simulink model "Force_Jawwad"  (R2023a)
settings: Solver=VariableStepAuto  StartTime=0.0  StopTime=5  RelTol=1e-3
undefined symbols (not defined in the file): fd, Kd, Kf, Ki, Kp, Md, parms
settings Model: Creator=uzair  LastModifiedBy=syedj
settings OptimizationCC: ReuseModelBlockBuffer=off

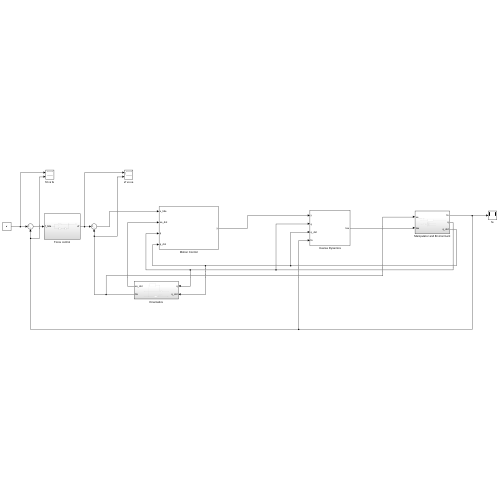
[thumbnail: Simulink's stored preview of the top-level diagram]
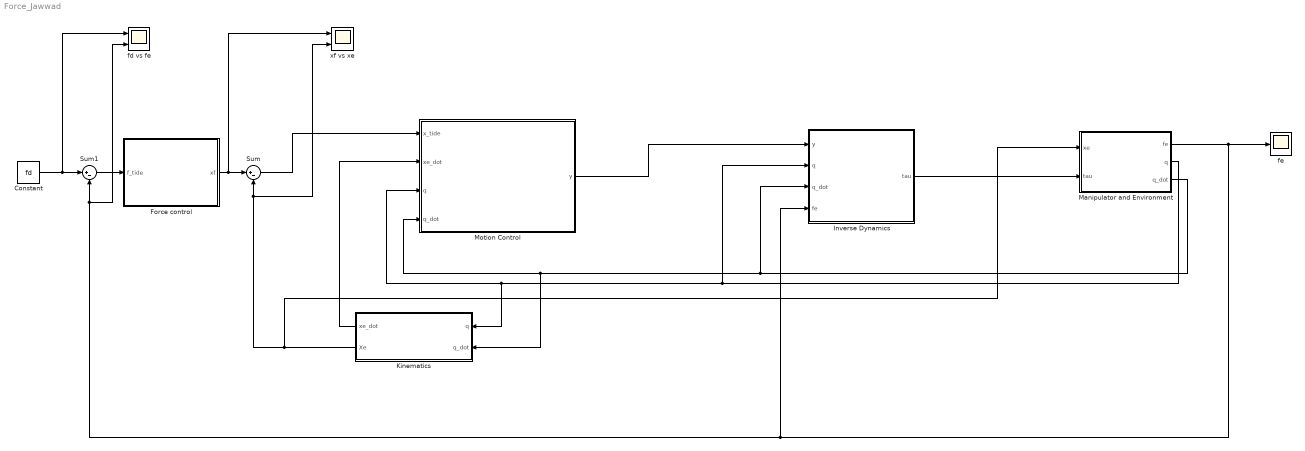
== system Force_Jawwad ==
  Constant : Constant  Value=fd
  Force control : Subsystem
  Inverse Dynamics : Subsystem
  Kinematics : Subsystem
  Manipulator and Environment : Subsystem
  Motion Control : Subsystem
  Sum : Sum  Inputs=|+-
  Sum1 : Sum  Inputs=|+-
  fd vs fe : Scope  NumInputPorts=2
  fe : Scope
  xf vs xe : Scope  NumInputPorts=2
  wires:
  Motion Control/1(y) -> Inverse Dynamics/1(y)
  Kinematics/2(Xe) -> xf vs xe/2, Sum/2, Manipulator and Environment/1(xe)
  Kinematics/1(xe_dot) -> Motion Control/2(xe_dot)
  Manipulator and Environment/2(q) -> Inverse Dynamics/2(q), Kinematics/1(q), Motion Control/3(q)
  Manipulator and Environment/3(q_dot) -> Inverse Dynamics/3(q_dot), Kinematics/2(q_dot), Motion Control/4(q_dot)
  Manipulator and Environment/1(fe) -> fe/1, Sum1/2, fd vs fe/2, Inverse Dynamics/4(fe)
  Inverse Dynamics/1(tau) -> Manipulator and Environment/2(tau)
  Sum/1 -> Motion Control/1(x_tide)
  Force control/1(xf) -> xf vs xe/1, Sum/1
  Constant/1 -> fd vs fe/1, Sum1/1
  Sum1/1 -> Force control/1(f_tide)

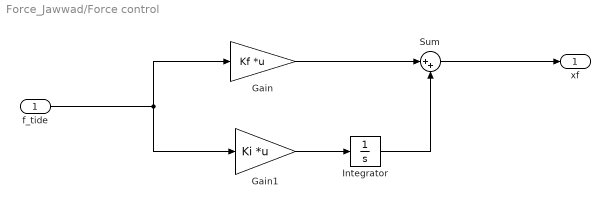
== system Force_Jawwad/Force control ==
  f_tide : Inport
  Gain : Gain  Gain=Kf  Multiplication=Matrix(K*u)
  Gain1 : Gain  Gain=Ki  Multiplication=Matrix(K*u)
  Integrator : Integrator
  Sum : Sum  Inputs=|++
  xf : Outport
  wires:
  f_tide/1 -> Gain1/1, Gain/1
  Gain1/1 -> Integrator/1
  Integrator/1 -> Sum/2
  Gain/1 -> Sum/1
  Sum/1 -> xf/1

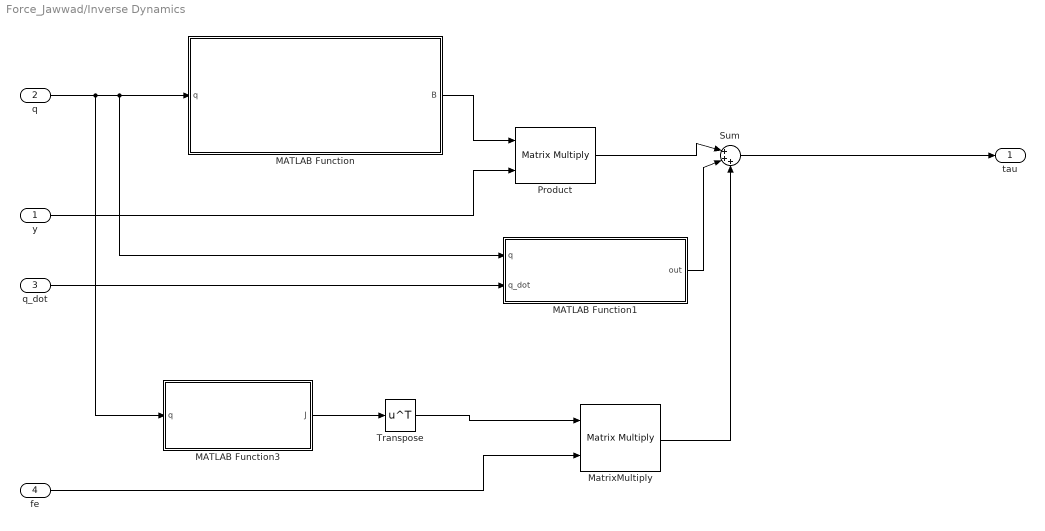
== system Force_Jawwad/Inverse Dynamics ==
  y : Inport
  q : Inport  Port=2
  q_dot : Inport  Port=3
  fe : Inport  Port=4
  MATLAB Function : MATLAB Function  TreatAsAtomicUnit=on
  MATLAB Function1 : MATLAB Function  TreatAsAtomicUnit=on
  MATLAB Function3 : MATLAB Function  TreatAsAtomicUnit=on
  MatrixMultiply : Product  Multiplication=Matrix(*)
  Product : Product  Multiplication=Matrix(*)
  Sum : Sum  Inputs=|+++
  Transpose : Math  Operator=transpose  OutputSignalType=real
  tau : Outport
  wires:
  q/1 -> MATLAB Function3/1(q), MATLAB Function1/1(q), MATLAB Function/1(q)
  MATLAB Function/1(B) -> Product/1
  y/1 -> Product/2
  q_dot/1 -> MATLAB Function1/2(q_dot)
  MATLAB Function1/1(out) -> Sum/2
  Sum/1 -> tau/1
  MATLAB Function3/1(J) -> Transpose/1
  fe/1 -> MatrixMultiply/2
  Transpose/1 -> MatrixMultiply/1
  MatrixMultiply/1 -> Sum/3
  Product/1 -> Sum/1

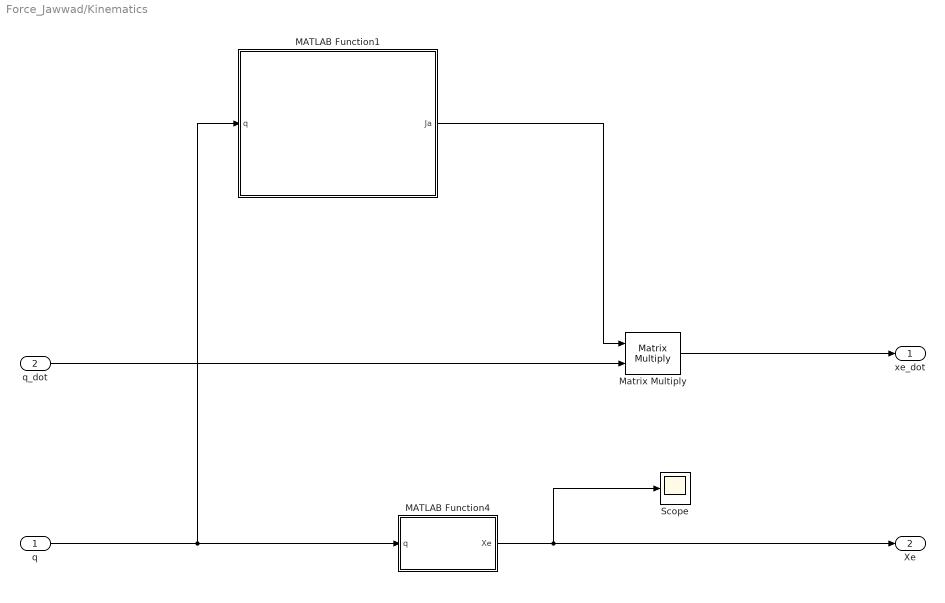
== system Force_Jawwad/Kinematics ==
  q : Inport
  q_dot : Inport  Port=2
  MATLAB Function1 : MATLAB Function  TreatAsAtomicUnit=on
  MATLAB Function4 : MATLAB Function  TreatAsAtomicUnit=on
  Matrix Multiply : Product  Multiplication=Matrix(*)
  Scope : Scope
  xe_dot : Outport
  Xe : Outport  Port=2
  wires:
  MATLAB Function1/1(Ja) -> Matrix Multiply/1
  q/1 -> MATLAB Function1/1(q), MATLAB Function4/1(q)
  MATLAB Function4/1(Xe) -> Scope/1, Xe/1
  Matrix Multiply/1 -> xe_dot/1
  q_dot/1 -> Matrix Multiply/2

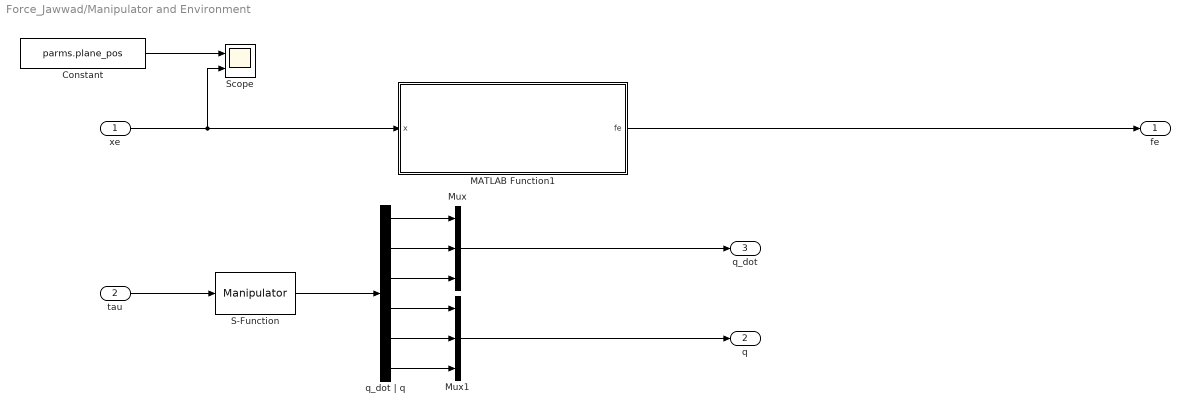
== system Force_Jawwad/Manipulator and Environment ==
  xe : Inport
  tau : Inport  Port=2
  Constant : Constant  Value=parms.plane_pos
  MATLAB Function1 : MATLAB Function  TreatAsAtomicUnit=on
  Mux : Mux  Inputs=3
  Mux1 : Mux  Inputs=3
  S-Function : S-Function  FunctionName=Manipulator  Parameters=params  SFunctionDeploymentMode=off  EnableBusSupport=off
  Scope : Scope  NumInputPorts=2
  q_dot | q : Demux  Outputs=6
  fe : Outport
  q : Outport  Port=2
  q_dot : Outport  Port=3
  wires:
  MATLAB Function1/1(fe) -> fe/1
  S-Function/1 -> q_dot | q/1
  q_dot | q/4 -> Mux1/1
  q_dot | q/1 -> Mux/1
  q_dot | q/6 -> Mux1/3
  q_dot | q/2 -> Mux/2
  q_dot | q/5 -> Mux1/2
  q_dot | q/3 -> Mux/3
  Mux/1 -> q_dot/1
  Mux1/1 -> q/1
  tau/1 -> S-Function/1
  Constant/1 -> Scope/1
  xe/1 -> Scope/2, MATLAB Function1/1(x)

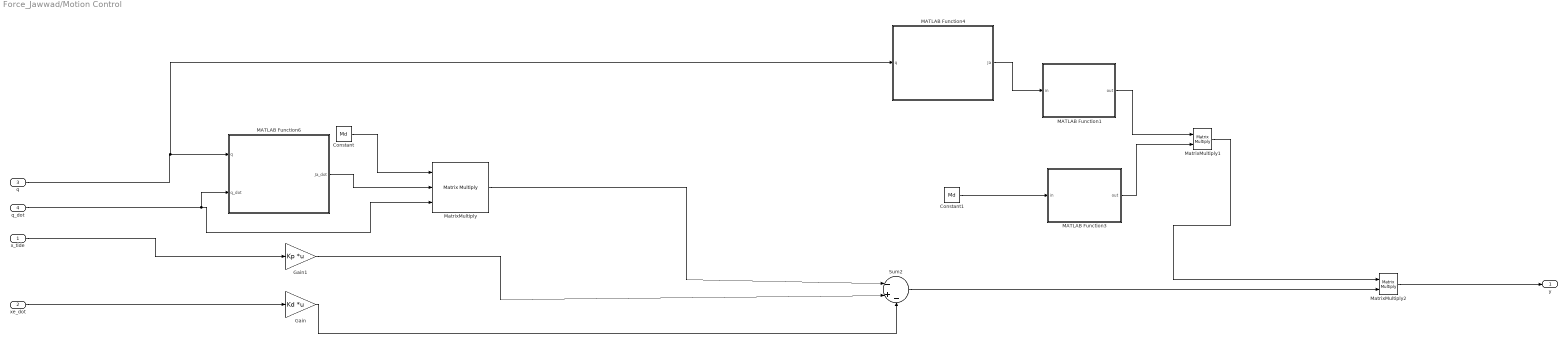
== system Force_Jawwad/Motion Control ==
  x_tide : Inport
  xe_dot : Inport  Port=2
  q : Inport  Port=3
  q_dot : Inport  Port=4
  Constant : Constant  Value=Md  VectorParams1D=off
  Constant1 : Constant  Value=Md  VectorParams1D=off
  Gain : Gain  Gain=Kd  Multiplication=Matrix(K*u)
  Gain1 : Gain  Gain=Kp  Multiplication=Matrix(K*u)
  MATLAB Function1 : MATLAB Function  TreatAsAtomicUnit=on
  MATLAB Function3 : MATLAB Function  TreatAsAtomicUnit=on
  MATLAB Function4 : MATLAB Function  TreatAsAtomicUnit=on
  MATLAB Function6 : MATLAB Function  TreatAsAtomicUnit=on
  MatrixMultiply : Product  Inputs=3  Multiplication=Matrix(*)
  MatrixMultiply1 : Product  Multiplication=Matrix(*)
  MatrixMultiply2 : Product  Multiplication=Matrix(*)
  Sum2 : Sum  Inputs=|-+-
  y : Outport
  wires:
  q/1 -> MATLAB Function4/1(q), MATLAB Function6/1(q)
  q_dot/1 -> MATLAB Function6/2(q_dot), MatrixMultiply/3
  Constant/1 -> MatrixMultiply/1
  MATLAB Function6/1(Ja_dot) -> MatrixMultiply/2
  MATLAB Function1/1(out) -> MatrixMultiply1/1
  MATLAB Function3/1(out) -> MatrixMultiply1/2
  MATLAB Function4/1(Ja) -> MATLAB Function1/1(in)
  Constant1/1 -> MATLAB Function3/1(in)
  Sum2/1 -> MatrixMultiply2/2
  MatrixMultiply1/1 -> MatrixMultiply2/1
  MatrixMultiply2/1 -> y/1
  xe_dot/1 -> Gain/1
  x_tide/1 -> Gain1/1
  MatrixMultiply/1 -> Sum2/1
  Gain/1 -> Sum2/3
  Gain1/1 -> Sum2/2

== matlab function Force_Jawwad/Inverse Dynamics/MATLAB Function1 ==
  data: q input; out output; q_dot input; params parameter
function out = n(q, q_dot, params)
    
    m1 = params.m(1);
    m2 = params.m(2);
    m3 = params.m(3);

    q1 = q(1);
    q2 = q(2);
    q3 = q(3);

    q1_dot = q_dot(1);
    q2_dot = q_dot(2);
    q3_dot = q_dot(3);
    
    r1 = 0.4;
    a1 = 0.02;
    a2 = 0.03;
    a3 = 0.01;
    b1 = 0.1256;
    b2 = 0.03;
    b3 = 0.01;
    c1 = 0.4;
    c2 = 0.46;
    c3 = 0.15;
    g = params.g;

    Fv = params.Fv;
 

   C = [[ (m3*q3_dot*(2*c1 + c3 + 2*q3))/2, 0, (m3*q1_dot*(2*c1 + c3 + 2*q3))/2]
[                                0, 0,                                0]
[-(m3*q1_dot*(2*c1 + c3 + 2*q3))/2, 0,                                0]];

G = [(c1*g*m1*cos(q1))/2 + g*m2*cos(q1)*(c1 - c2/2) + g*m3*cos(q1)*(c1 + c3/2 + q3)
        0;
        g*m3*sin(q1)];
out = C*q_dot + diag(Fv)*q_dot + G;
end

== matlab function Force_Jawwad/Inverse Dynamics/MATLAB Function ==
  data: q input; B output; params parameter
function B = inertiaMatrix(q, params)
    q1 = q(1); % not used in this matrix
    q2 = q(2);
    q3 = q(3);

    m1 = params.m(1);
    m2 = params.m(2);
    m3 = params.m(3);
        
    r1 = 0.4;
    a1 = 0.02;
    a2 = 0.03;
    a3 = 0.01;
    b1 = 0.1256;
    b2 = 0.03;
    b3 = 0.01;
    c1 = 0.4;
    c2 = 0.46;
    c3 = 0.15;

   B = [[(a2^2*m2)/12 + (3*a1^4*m1)/2 + (a3^2*m3)/12 + (3*b1^4*m1)/2 + (b3^2*m3)/12 + c1^2*m1 + c1^2*m2 + c1^2*m3 + (7*c2^2*m2)/12 + (c3^2*m3)/2 + m3*q3^2 + 3*a1^2*b1^2*m1 - c1*c2*m2 + c1*c3*m3 + 2*c1*m3*q3 + c3*m3*q3,       0,  0]
[                                                                                                                                                                                                               0, m2 + m3,  0]
[                                                                                                                                                                                                               0,       0, m3]];
end

== matlab function Force_Jawwad/Kinematics/MATLAB Function4 ==
  data: q input; Xe output
function Xe = Kinematics(q)
    q1 = q(1);
    q2 = q(2);
    q3 = q(3);
     
    r1 = 0.4;
    a1 = 0.02;
    a2 = 0.03;
    a3 = 0.01;
    b1 = 0.1256;
    b2 = 0.03;
    b3 = 0.01;
    c1 = 0.4;
    c2 = 0.46;
    c3 = 0.15;
    
    H = [[0, -sin(q1), cos(q1),              cos(q1)*(c1 + c3 + q3)]
[1,        0,       0,                           - c2 - q2]
[0,  cos(q1), sin(q1), r1 + sin(q1)*(c3 + q3) + c1*sin(q1)]
[0,        0,       0,                                   1]];


    eulers = rotm2eul(H(1:3,1:3), "ZYZ");

    Xe = [H(1:3,4)];
end

== matlab function Force_Jawwad/Motion Control/MATLAB Function1 ==
  data: in input; out output
function out = inv(in)
    out = pinv(in);
end

== matlab function Force_Jawwad/Kinematics/MATLAB Function1 ==
  data: q input; Ja output
function Ja = AnalyticalJacobian(q)
    
    q1 = q(1);
    q2 = q(2);
    q3 = q(3);
    
    r1 = 0.4;
    a1 = 0.02;
    a2 = 0.03;
    a3 = 0.01;
    b1 = 0.1256;
    b2 = 0.03;
    b3 = 0.01;
    c1 = 0.4;
    c2 = 0.46;
    c3 = 0.15;

       H = [[0, -sin(q1), cos(q1),              cos(q1)*(c1 + c3 + q3)]
[1,        0,       0,                           - c2 - q2]
[0,  cos(q1), sin(q1), r1 + sin(q1)*(c3 + q3) + c1*sin(q1)]
[0,        0,       0,                                   1]];


        eulers = rotm2eul(H(1:3,1:3), "ZYZ");


        phi1 = eulers(1);
        phi2 = eulers(2);
        phi3 = eulers(3); %not used

        
Ja_m = [
[        -sin(q1)*(c1 + c3 + q3),  0, cos(q1)]
[                              0, -1,       0]
[         cos(q1)*(c1 + c3 + q3),  0, sin(q1)]
];

Ja = Ja_m;

end

== matlab function Force_Jawwad/Manipulator and Environment/MATLAB Function1 ==
  data: x input; fe output; parms parameter
function fe = Environment(x, parms)
    if(x(parms.plane_axis) >= parms.plane_pos(parms.plane_axis))
        xr = parms.plane_pos;

        xe = zeros(3,1);
        xe(parms.plane_axis) = x(parms.plane_axis);

        fe = parms.Ke * (xe - xr);

    else
        fe = zeros(3,1);
    end
end

== matlab function Force_Jawwad/Motion Control/MATLAB Function3 ==
  data: in input; out output
function out = inv(in)
    out = pinv(in);
end

== matlab function Force_Jawwad/Motion Control/MATLAB Function4 ==
  data: q input; Ja output
function Ja = AnalyticalJacobian(q)
    
    q1 = q(1);
    q2 = q(2);
    q3 = q(3);
    
    r1 = 0.4;
    a1 = 0.02;
    a2 = 0.03;
    a3 = 0.01;
    b1 = 0.1256;
    b2 = 0.03;
    b3 = 0.01;
    c1 = 0.4;
    c2 = 0.46;
    c3 = 0.15;

       H = [[0, -sin(q1), cos(q1),              cos(q1)*(c1 + c3 + q3)]
[1,        0,       0,                           - c2 - q2]
[0,  cos(q1), sin(q1), r1 + sin(q1)*(c3 + q3) + c1*sin(q1)]
[0,        0,       0,                                   1]];


        eulers = rotm2eul(H(1:3,1:3), "ZYZ");


        phi1 = eulers(1);
        phi2 = eulers(2);
        phi3 = eulers(3); %not used

        
Ja_m = [
[        -sin(q1)*(c1 + c3 + q3),  0, cos(q1)]
[                              0, -1,       0]
[         cos(q1)*(c1 + c3 + q3),  0, sin(q1)]
];

Ja = Ja_m;

end

== matlab function Force_Jawwad/Inverse Dynamics/MATLAB Function3 ==
  data: q input; J output
function J = GeomatricalJacobian(q)
q1 = q(1);
q2 = q(2);
q3 = q(3);
   
    r1 = 0.4;
    a1 = 0.02;
    a2 = 0.03;
    a3 = 0.01;
    b1 = 0.1256;
    b2 = 0.03;
    b3 = 0.01;
    c1 = 0.4;
    c2 = 0.46;
    c3 = 0.15;

    J = [
[-sin(q1)*(c1 + c3 + q3),  0, cos(q1)]
[                      0, -1,       0]
[ cos(q1)*(c1 + c3 + q3),  0, sin(q1)]
];

end

== matlab function Force_Jawwad/Motion Control/MATLAB Function6 ==
  data: q input; Ja_dot output; q_dot input
function Ja_dot = AnalyticalJacobian_Dot(q, q_dot)
q1 = q(1);
q2 = q(2);
q3 = q(3);

    r1 = 0.4;
    a1 = 0.02;
    a2 = 0.03;
    a3 = 0.01;
    b1 = 0.1256;
    b2 = 0.03;
    b3 = 0.01;
    c1 = 0.4;
    c2 = 0.46;
    c3 = 0.15;

q1_dot = q_dot(1);
q2_dot = q_dot(2);
q3_dot = q_dot(3);

H = [[0, -sin(q1), cos(q1),              cos(q1)*(c1 + c3 + q3)]
[1,        0,       0,                           - c2 - q2]
[0,  cos(q1), sin(q1), r1 + sin(q1)*(c3 + q3) + c1*sin(q1)]];



eulers = rotm2eul(H(1:3,1:3), "ZYZ");


phi1 = eulers(1);
phi2 = eulers(2);
phi3 = eulers(3); %not used

Ja_dot_m = [
[        -cos(q1)*q1_dot*(c1 + c3 + q3)-sin(q1)*q3_dot,  0, -sin(q1)*q1_dot]
[                              0, 0,       0]
[         -sin(q1)*q1_dot*(c1 + c3 + q3)+cos(q1)*q3_dot,  0, cos(q1)*q1_dot]
];

Ja_dot = Ja_dot_m;
end
